simulink model "problem7_ReferenceModel"  (R2020b)
settings: Solver=FixedStepAuto  StartTime=0.0  StopTime=10.0  FixedStep=0.2  RelTol=1e-3
settings Model: Creator=admin  LastModifiedBy=admin
settings DataIOCC: SaveOutput=off  SaveTime=off

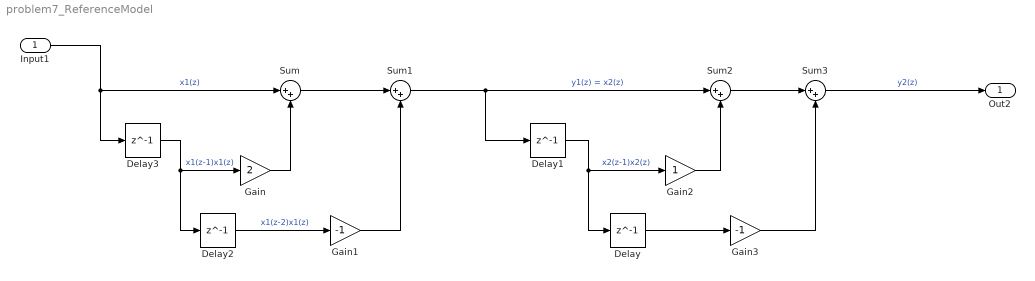
== system problem7_ReferenceModel ==
  Input1 : Inport  OutDataTypeStr=double  PortDimensions=1  SampleTime=[0.20000000000000001,0]
  Delay{,1..3} (4 alike) : Delay  DelayLength=1
  Gain : Gain  Gain=2
  Gain1 : Gain  Gain=-1
  Gain2 : Gain
  Gain3 : Gain  Gain=-1
  Sum{,1..3} (4 alike) : Sum  Inputs=|++
  Out2 : Outport  OutDataTypeStr=double  PortDimensions=1  SampleTime=[0.20000000000000001,0]
  wires:
  Delay1/1 -> Gain2/1, Delay/1  "x2(z-1)x2(z)"
  Sum2/1 -> Sum3/1
  Sum/1 -> Sum1/1
  Input1/1 -> Sum/1, Delay3/1  "x1(z)"
  Gain/1 -> Sum/2
  Delay3/1 -> Gain/1, Delay2/1  "x1(z-1)x1(z)"
  Sum1/1 -> Sum2/1, Delay1/1  "y1(z) = x2(z)"
  Gain1/1 -> Sum1/2
  Delay/1 -> Gain3/1
  Sum3/1 -> Out2/1  "y2(z)"
  Delay2/1 -> Gain1/1  "x1(z-2)x1(z)"
  Gain3/1 -> Sum3/2
  Gain2/1 -> Sum2/2
